simulink model "Lecture10_11Exercise"  (R2020b)
settings: Solver=VariableStepAuto  StartTime=0.0  StopTime=10  RelTol=1e-3
values from neighbouring files (symbols this model uses):
  A = [-Ra/La -Ka/La; Ka/J -B/J]    [Lecture10_11Exercise.m]    (also in Lecture5Exercises.m = [2.7 0.8 0.7; 1 0 0; 0 1 0]; Lecture6Exercise.m = [0 1 0; 0 -B/J Ka/J; 0 -Km/La -Ra/La]; Lecture7Exercise.m = [0, 1; -1, -2])
  A_aa = A_adj(1,1)    [Lecture10_11Exercise.m]    (also in Lecture5Exercises.m)
  A_ab = A_adj(1,2)    [Lecture10_11Exercise.m]    (also in Lecture5Exercises.m = [A_adj(1,2) A_adj(1,3)])
  A_ba = A_adj(2,1)    [Lecture10_11Exercise.m]    (also in Lecture5Exercises.m = [A_adj(2,1); A_adj(3,1)])
  A_bb = A_adj(2,2)    [Lecture10_11Exercise.m]    (also in Lecture5Exercises.m = [A_adj(2,2) A_adj(2,3); A_adj(3,2) A_adj(3,3)])
  Ad = [0.8, -0.36; 0.09, 0.98]    [Lecture4Exercise.m]
  B = [1/La;0]    [Lecture10_11Exercise.m]    (also in Lecture5Exercises.m = [1; 0; 0]; Lecture6Exercise.m = [0; 0; 1/La]; Lecture7Exercise.m = [0; 1])
  B_a = B_adj(1)    [Lecture10_11Exercise.m]    (also in Lecture5Exercises.m)
  B_b = B_adj(2)    [Lecture10_11Exercise.m]    (also in Lecture5Exercises.m = [B_adj(2); B_adj(3)])
  Bd = [0.09; 0.0047]    [Lecture4Exercise.m]
  C = [0 1]    [Lecture10_11Exercise.m]    (also in Lecture5Exercises.m = [0 0 1]; Lecture6Exercise.m = [1 0 0]; Lecture7Exercise.m = [1, 0])
  C_adj = [Cd(2) Cd(1)]    [Lecture10_11Exercise.m]    (also in Lecture5Exercises.m = [Cd(3) Cd(2) Cd(1)])
  Cd = C    [Lecture10_11Exercise.m]    (also in Lecture4Exercise.m = [0, 10]; Lecture5Exercises.m; Lecture6Exercise.m)
  D_analog = tf(Kp*Ki*[tau_i 1], [tau_i 0])    [Lecture10_11Exercise.m]
  D_digital_z = c2d(D_digital_w, T)    [Lecture10_11Exercise.m]
  Gs = tf(10, [1 3 0])    [Assignment3.m]    (also in Lecture10_11Exercise.m = tf(num,den); Lecture3Exercise.m = tf(10, [1 2 0]); Lecture5Exercises.m = tf([4], [1 2 4 4]); Lecture6Exercise.m = tf(num,den))
  K_s = KKi_s(1:n-1)    [Lecture10_11Exercise.m]
  K_z = acker(A_adj, B_adj, [z_p_plant, z_p_plant])    [Lecture10_11Exercise.m]
  Kd = 9 - 3/2    (= 7.5)    [Lecture10_11Exercise.m]    (also in Lecture3Exercise.m = 0.4)
  Ki = 27    [Lecture10_11Exercise.m]    (also in Lecture4Exercise.m = -KKi(3))
  Ki_s = -KKi_s(n)    [Lecture10_11Exercise.m]
  Ki_z = -KKi_z(n)    [Lecture10_11Exercise.m]
  Kp = 27 - 3/5    (= 26.4)    [Lecture10_11Exercise.m]    (also in Lecture3Exercise.m = 0.9)
  L = acker(A_bb', A_ab', z_p_obs)'    [Lecture10_11Exercise.m]    (also in Lecture1Pendulum.m = 1; Lecture5Exercises.m = acker(A_bb', A_ab', [zper zper])')
  T = 0.1    [Lecture10_11Exercise.m]    (also in Lecture4Exercise.m)
settings Model: Creator=sebastian  LastModifiedBy=sebastian

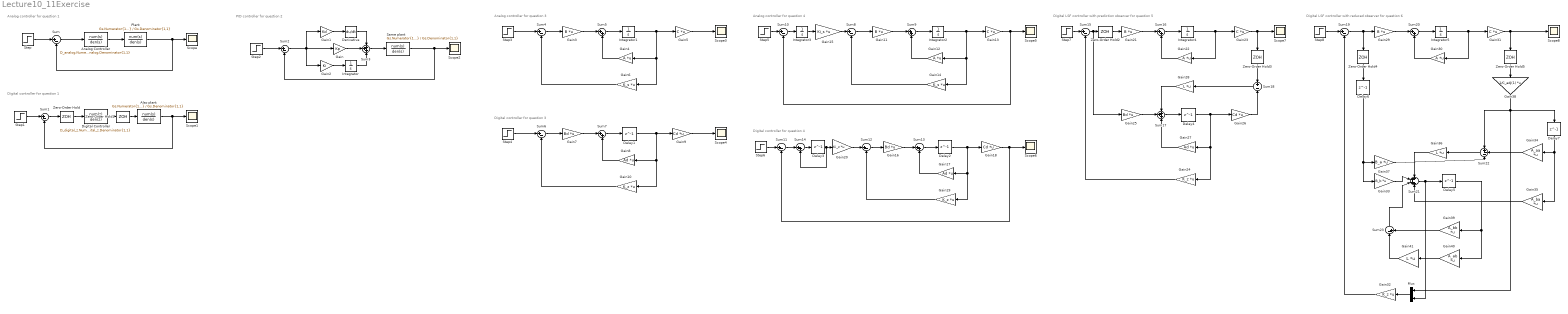
== system Lecture10_11Exercise ==
  note: Analog controller for question 3
  note: Analog controller for question 1
  note: Digital controller for question 1
  note: PID controller for question 2
  note: Digital controller for question 3
  note: Analog controller for question 4
  note: Digital controller for question 4
  note: Digital LSF controller with prediction observer for question 5
  note: Digital LSF controller with reduced observer for question 6
  Also plant : TransferFcn  Numerator=Gs.Numerator{1,1}  Denominator=Gs.Denominator{1,1}
  Analog Controller : TransferFcn  Numerator=D_analog.Numerator{1,1}  Denominator=D_analog.Denominator{1,1}
  Delay{1..7} (7 alike) : Delay  DelayLength=1  SampleTime=T
  Derivative : Derivative
  Digital Controller : DiscreteTransferFcn  Numerator=D_digital_z.Numerator{1,1}  Denominator=D_digital_z.Denominator{1,1}  SampleTime=T
  Gain : Gain  Gain=Kp
  Gain1 : Gain  Gain=Kd
  Gain{10,19,24,32} (4 alike) : Gain  Gain=K_z  Multiplication=Matrix(K*u)
  Gain{3,11,21,29} (4 alike) : Gain  Gain=B  Multiplication=Matrix(K*u)
  Gain{4,12,22,30} (4 alike) : Gain  Gain=A  Multiplication=Matrix(K*u)
  Gain{5,13,23,31} (4 alike) : Gain  Gain=C  Multiplication=Matrix(K*u)
  Gain14 : Gain  Gain=K_s  Multiplication=Matrix(K*u)
  Gain15 : Gain  Gain=Ki_s  Multiplication=Matrix(K*u)
  Gain16 : Gain  Gain=Bd  Multiplication=Matrix(K*u)
  Gain17 : Gain  Gain=Ad  Multiplication=Matrix(K*u)
  Gain18 : Gain  Gain=Cd  Multiplication=Matrix(K*u)
  Gain2 : Gain  Gain=Ki
  Gain20 : Gain  Gain=Ki_z  Multiplication=Matrix(K*u)
  Gain25 : Gain  Gain=Bd  Multiplication=Matrix(K*u)
  Gain26 : Gain  Gain=Cd  Multiplication=Matrix(K*u)
  Gain27 : Gain  Gain=Ad  Multiplication=Matrix(K*u)
  Gain28 : Gain  Gain=L  Multiplication=Matrix(K*u)
  Gain33 : Gain  Gain=B_b  Multiplication=Matrix(K*u)
  Gain34 : Gain  Gain=A_aa  Multiplication=Matrix(K*u)
  Gain35 : Gain  Gain=A_ba  Multiplication=Matrix(K*u)
  Gain36 : Gain  Gain=L  Multiplication=Matrix(K*u)
  Gain37 : Gain  Gain=B_a  Multiplication=Matrix(K*u)
  Gain38 : Gain  Gain=1/C_adj(1)  Multiplication=Matrix(K*u)
  Gain39 : Gain  Gain=A_bb  Multiplication=Matrix(K*u)
  Gain40 : Gain  Gain=A_ab  Multiplication=Matrix(K*u)
  Gain41 : Gain  Gain=L  Multiplication=Matrix(K*u)
  Gain6 : Gain  Gain=K_s  Multiplication=Matrix(K*u)
  Gain7 : Gain  Gain=Bd  Multiplication=Matrix(K*u)
  Gain8 : Gain  Gain=Ad  Multiplication=Matrix(K*u)
  Gain9 : Gain  Gain=Cd  Multiplication=Matrix(K*u)
  Integrator{,1..5} (6 alike) : Integrator
  Mux : Mux  Inputs=2
  Plant : TransferFcn  Numerator=Gs.Numerator{1,1}  Denominator=Gs.Denominator{1,1}
  Same plant : TransferFcn  Numerator=Gs.Numerator{1,1}  Denominator=Gs.Denominator{1,1}
  Scope{,1..8} (9 alike) : Scope
  Step{,1..8} (9 alike) : Step  SampleTime=0
  Sum{,1..2,4,6,8,10..12,15,19} (11 alike) : Sum  Inputs=|+-
  Sum{5,7,9,13..14,16,20} (7 alike) : Sum  Inputs=|++
  Sum17 : Sum  Inputs=+++
  Sum18 : Sum  Inputs=+|-
  Sum21 : Sum  Inputs=++++
  Sum22 : Sum  Inputs=+--
  Sum23 : Sum  Inputs=|-+
  Sum3 : Sum  Inputs=+++
  Zero-Order Hold{,1..5} (6 alike) : ZeroOrderHold  SampleTime=T
  wires:
  Step/1 -> Sum/1
  Plant/1 -> Sum/2, Scope/1
  Sum/1 -> Analog Controller/1
  Analog Controller/1 -> Plant/1
  Also plant/1 -> Sum1/2, Scope1/1
  Sum1/1 -> Zero-Order Hold/1
  Step1/1 -> Sum1/1
  Digital Controller/1 -> Zero-Order Hold1/1
  Zero-Order Hold/1 -> Digital Controller/1
  Zero-Order Hold1/1 -> Also plant/1
  Same plant/1 -> Sum2/2, Scope2/1
  Sum2/1 -> Gain1/1, Gain2/1, Gain/1
  Step2/1 -> Sum2/1
  Sum3/1 -> Same plant/1
  Gain/1 -> Sum3/2
  Gain2/1 -> Integrator/1
  Integrator/1 -> Sum3/3
  Gain1/1 -> Derivative/1
  Derivative/1 -> Sum3/1
  Step3/1 -> Sum4/1
  Sum4/1 -> Gain3/1
  Gain3/1 -> Sum5/1
  Gain4/1 -> Sum5/2
  Sum5/1 -> Integrator1/1
  Integrator1/1 -> Gain5/1, Gain6/1, Gain4/1
  Gain5/1 -> Scope3/1
  Gain6/1 -> Sum4/2
  Gain8/1 -> Sum7/2
  Gain9/1 -> Scope4/1
  Step4/1 -> Sum6/1
  Gain10/1 -> Sum6/2
  Sum7/1 -> Delay1/1
  Sum6/1 -> Gain7/1
  Delay1/1 -> Gain9/1, Gain10/1, Gain8/1
  Gain7/1 -> Sum7/1
  Gain12/1 -> Sum9/2
  Gain13/1 -> Sum10/2, Scope5/1
  Sum8/1 -> Gain11/1
  Gain14/1 -> Sum8/2
  Sum9/1 -> Integrator2/1
  Integrator2/1 -> Gain13/1, Gain14/1, Gain12/1
  Gain11/1 -> Sum9/1
  Step5/1 -> Sum10/1
  Sum10/1 -> Integrator3/1
  Integrator3/1 -> Gain15/1
  Gain15/1 -> Sum8/1
  Gain16/1 -> Sum13/1
  Delay3/1 -> Sum14/2, Gain20/1
  Delay2/1 -> Gain18/1, Gain19/1, Gain17/1
  Gain20/1 -> Sum12/1
  Sum11/1 -> Sum14/1
  Gain19/1 -> Sum12/2
  Step6/1 -> Sum11/1
  Sum12/1 -> Gain16/1
  Gain17/1 -> Sum13/2
  Gain18/1 -> Scope6/1, Sum11/2
  Sum13/1 -> Delay2/1
  Sum14/1 -> Delay3/1
  Gain22/1 -> Sum16/2
  Gain23/1 -> Zero-Order Hold3/1, Scope7/1
  Step7/1 -> Sum15/1
  Gain24/1 -> Sum15/2
  Sum16/1 -> Integrator4/1
  Integrator4/1 -> Gain23/1, Gain22/1
  Gain21/1 -> Sum16/1
  Gain25/1 -> Sum17/2
  Sum17/1 -> Delay4/1
  Delay4/1 -> Gain24/1, Gain27/1, Gain26/1
  Gain27/1 -> Sum17/3
  Gain26/1 -> Sum18/2
  Sum18/1 -> Gain28/1
  Gain28/1 -> Sum17/1
  Gain36/1 -> Sum21/1
  Sum19/1 -> Gain29/1, Zero-Order Hold4/1
  Integrator5/1 -> Gain31/1, Gain30/1
  Sum20/1 -> Integrator5/1
  Gain30/1 -> Sum20/2
  Sum21/1 -> Mux/2, Delay5/1
  Gain32/1 -> Sum19/2
  Sum22/1 -> Gain36/1
  Gain29/1 -> Sum20/1
  Step8/1 -> Sum19/1
  Gain31/1 -> Zero-Order Hold5/1, Scope8/1
  Sum15/1 -> Zero-Order Hold2/1, Gain25/1
  Zero-Order Hold3/1 -> Sum18/1
  Zero-Order Hold4/1 -> Delay6/1
  Delay6/1 -> Gain37/1, Gain33/1
  Zero-Order Hold5/1 -> Gain38/1
  Mux/1 -> Gain32/1
  Gain38/1 -> Mux/1, Sum22/1, Delay7/1
  Gain33/1 -> Sum21/2
  Delay7/1 -> Gain35/1, Gain34/1
  Gain35/1 -> Sum21/4
  Gain37/1 -> Sum22/3
  Gain34/1 -> Sum22/2
  Gain40/1 -> Gain41/1
  Gain41/1 -> Sum23/1
  Gain39/1 -> Sum23/2
  Sum23/1 -> Sum21/3
  Delay5/1 -> Gain40/1, Gain39/1
  Zero-Order Hold2/1 -> Gain21/1
